simulink subsystem "EnergyCalc"  (R2021b)
settings: Solver=VariableStepAuto  StartTime=0.0  StopTime=10.0  RelTol=1e-3
values from neighbouring files (symbols this model uses):
  Iwf = 0.2    [VehicleParams20_ver230707.m]
  Iwr = 0.2    [VehicleParams20_ver230707.m]
  M = 200+60    (= 260)    [VehicleParams20_ver230707.m]
settings Model: Creator=tsuyoshi  LastModifiedBy=tsuyoshi

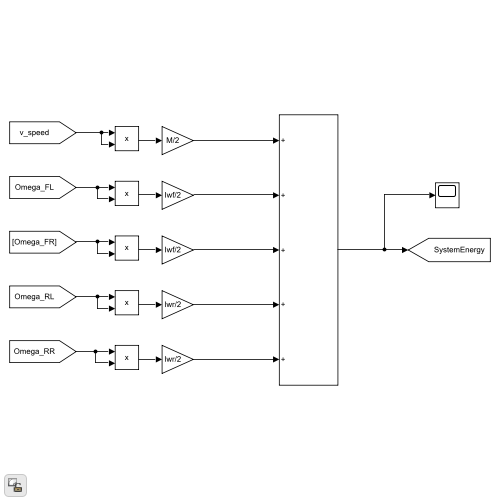
[thumbnail: Simulink's stored preview of the top-level diagram]
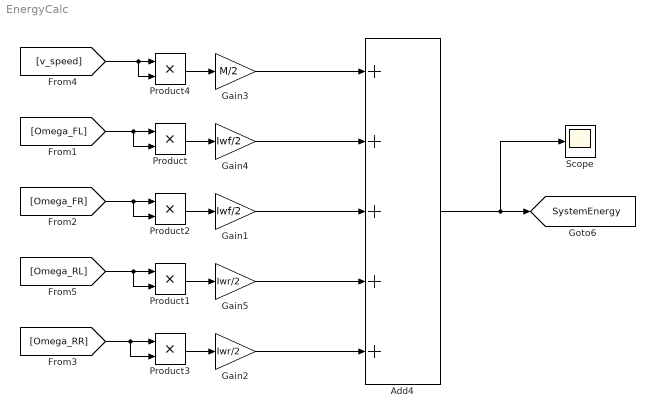
== system EnergyCalc ==
  Add4 : Sum  Inputs=+++++
  Gain1 : Gain  Gain=Iwf/2
  Gain2 : Gain  Gain=Iwr/2
  Gain3 : Gain  Gain=M/2
  Gain4 : Gain  Gain=Iwf/2
  Gain5 : Gain  Gain=Iwr/2
  Product{,1..4} (5 alike) : Product
  Scope : Scope
  tag scope: SystemEnergy=global
  wires:
  [Omega_FL] -> Product/1, Product/2
  Product/1 -> Gain4/1
  Add4/1 -> [SystemEnergy], Scope/1
  Gain4/1 -> Add4/2
  Gain5/1 -> Add4/4
  [Omega_RL] -> Product1/2, Product1/1
  Product1/1 -> Gain5/1
  Product2/1 -> Gain1/1
  [Omega_FR] -> Product2/2, Product2/1
  Gain1/1 -> Add4/3
  Product3/1 -> Gain2/1
  [Omega_RR] -> Product3/2, Product3/1
  Gain2/1 -> Add4/5
  Product4/1 -> Gain3/1
  [v_speed] -> Product4/1, Product4/2
  Gain3/1 -> Add4/1
